simulink model "PrimAff"  (Simulink 6.1)
settings: Solver=FixedStepDiscrete  StartTime=0.00  StopTime=tstop-tstep+100  FixedStep=tstep  RelTol=1e-3
PreLoadFcn:
  | global tstep tstop stim amdepth pmdepth freq
  | global tim sig ram rpm
  | global thold sigma spk
InitFcn:
  | genstim;
StopFcn:
  | beg_dat = (100/tstep)+1;
  | spk = spk(beg_dat:end);
values from neighbouring files (symbols this model uses):
  sigma = str2double(get(h.edit_noise, 'String'))    [PrimAff_IntFire.m]
  thold = str2double(get(h.edit_thold, 'String'))    [PrimAff_IntFire.m]
  tstep = str2double(get(h.edit_sampper, 'String'))    [PrimAff_IntFire.m]
settings Model: LastModifiedBy=Bruce Carlson
settings DataIOCC: LimitDataPoints=off  SaveOutput=off  SaveTime=off  SignalLoggingName=sigsOut
settings DebuggingCC: UnconnectedInputMsg=none  UnconnectedOutputMsg=none  UnconnectedLineMsg=none
settings HardwareCC: TargetUnknown=on
settings GRTTargetCC: ModelReferenceCompliant=off  MatFileLogging=off

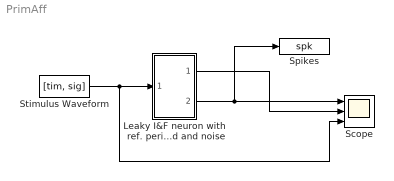
== system PrimAff ==
  Leaky I&F neuron with  ref. period and noise : Subsystem  mask(L I&F ref. per. noise){dt=tstep, thres=thold, sigma=sigma, C=0.1, R=10, ref=1}
      mask prompts: dt "time step [msec]"; thres "mean threshold [mV]"; sigma "noise st. dev."; C "Capacitance [nF]"; R "Resistance [MOhms]"; ref "refractory period [msec]"
      mask help: Parameters
      mask init:
      | if (ref<dt) disp(' '); disp('Warning: refractory period cannot be smaller than time step.'); disp(' '); end;
      mask Help: For a detailled description of the model, please type 'help liandfrn' in the main matlab window.
      mask Display: disp('Vm \n\n spikes')
  Scope : Scope  NumInputPorts=3
      settings: TickLabels=on  TimeRange=1000  YMin=-0.1~-50~-20  YMax=1.1~15~20  DataFormat=Array
  Spikes : ToWorkspace  VariableName=spk  SaveFormat=Array
      settings: MaxDataPoints=Inf
  Stimulus Waveform : FromWorkspace  VariableName=[tim, sig]  SampleTime=0  Interpolate=off  OutputAfterFinalValue=Holding final value
  wires:
  Stimulus Waveform/1 -> Scope/3, Leaky I&F neuron with  ref. period and noise/1(in_1)
  Leaky I&F neuron with  ref. period and noise/1(out_2) -> Scope/2
  Leaky I&F neuron with  ref. period and noise/2(out_1) -> Scope/1, Spikes/1

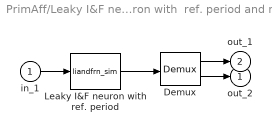
== system PrimAff/Leaky I&F neuron with  ref. period and noise ==
  in_1 : Inport  Port=1  LatchInput=off
  Demux : Demux  Outputs=2
  Leaky I&F neuron with ref. period : S-Function  FunctionName=liandfrn_sim  Parameters=dt,thres,sigma,C,R,ref
  out_2 : Outport  InitialOutput=0
  out_1 : Outport  Port=2  InitialOutput=0
  wires:
  Leaky I&F neuron with ref. period/1 -> Demux/1
  Demux/1 -> out_1/1
  Demux/2 -> out_2/1
  in_1/1 -> Leaky I&F neuron with ref. period/1
